simulink model "RIEKF_test"  (R2016b)
settings: Solver=ode23  StartTime=simulationParameters.startTime  StopTime=10  FixedStep=1e-5  EnableMultiTasking=on
InitFcn:
  | simulationInitFcn;
StartFcn:
  | simulationStartFcn;
StopFcn:
  | simulationStopFcn;
libraries: StateEstimation x1
settings Model: Creator=case  LastModifiedBy=Ross Hartley
settings SolverCC: EnableConcurrentExecution=on  ConcurrentTasks=on  ZeroCrossControl=DisableAll  InsertRTBMode=Always
settings DataIOCC: SaveOutput=off  SignalLogging=off  DSMLogging=off  SaveTime=off
settings OptimizationCC: DefaultParameterBehavior=Inlined  UseFloatMulNetSlope=on  InlineInvariantSignals=on  EfficientFloat2IntCast=on  LifeSpan=inf  SimCompilerOptimization=on  AccelVerboseBuild=on
settings DebuggingCC: ReadBeforeWriteMsg=DisableAll  WriteAfterWriteMsg=DisableAll  WriteAfterReadMsg=DisableAll  ParameterUnderflowMsg=error  ParameterTunabilityLossMsg=error  UniqueDataStoreMsg=error  AllowSymbolicDim=off  StrictBusMsg=ErrorOnBusTreatedAsVector  SFUnexpectedBacktrackingDiag=warning  SFNoUnconditionalDefaultTransitionDiag=warning  SFExecutionAtInitializationDiag=none
settings HardwareCC: TargetBitPerPointer=64  TargetBitPerSizeT=64  TargetBitPerPtrDiffT=64  TargetLongLongMode=on  TargetIntDivRoundTo=Zero  TargetEndianess=LittleEndian  TargetWordSize=64  TargetHWDeviceType=MATLAB Host  ProdEqTarget=off
settings ModelReferenceCC: UpdateModelReferenceTargets=IfOutOfDate  ModelReferenceNumInstancesAllowed=Zero  ModelReferenceMinAlgLoopOccurrences=on  PropagateSignalLabelsOutOfModel=off
settings RTWCC: RTWUseSimCustomCode=on  BuildConfiguration=Faster Runs  CheckMdlBeforeBuild=Warning
settings CodeAppCC: GenerateComments=off  SimulinkBlockComments=off
settings GRTTargetCC: MatFileLogging=off  MultiInstanceERTCode=on  CodeInterfacePackaging=Reusable function  SupportNonFinite=off  GenerateAllocFcn=on
settings ConfigComp: CovMetricSettings=dw  CovHtmlReporting=on  CovSaveCumulativeToWorkspaceVar=on  CovSaveSingleToWorkspaceVar=on  CovExternalEMLEnable=off
settings DiagnosticsConfigSet: SimMechanicsRigidlyBoundBlock=warning
settings ExplorerConfigSet: InternalSimMechanicsExplorerSettings="<ExplorerConfiguration><canonicalview>default</canonicalview><AnimationSetting><BasePlaybackSpeed>1.0</BasePlaybackSpeed><PlaybackSpeedFactor>1.0</PlaybackSpeedFactor></AnimationSetting><TilePanel><TileInfo><Tiles Columns=\"1\" Count=\"1\" Rows=\"1\"><Column Left=\"2\" Weight=\"1\"/><Column Left=\"1053\"/><Row Top=\"2\" Weight=\"1\"/><Row Top=\"486\"/><Tile Height=\"1\" Width=\"1\" X=\"0\" Y=\"0\"/></Tiles></TileInfo><SceneInfo><SceneViewer><BGColor><R>0.60000002384185791</R><G>0.60000002384185791</G><B>0.60000002384185791</B></BGColor><Camera><DoPerspective>on</DoPerspective><Position><X>1.5163613923952763</X><Y>-1.4988060678602755</Y><Z>0.66118837525886986</Z></Position><Center><X>0.016361392395276342</X><Y>0.0011939321397245184</Y><Z>0.16118837525886986</Z></Center><Up><X>0</X><Y>0</Y><Z>1</Z></Up><ViewLimDist>1</ViewLimDist><YLim>0.46630765815499858</YLim><XLim>1.0229317469421231</XLim></Camera></SceneViewer></SceneInfo></TilePanel><MechEditorPanel><Cameras><Camera><Id>Camera1</Id><Value><Name>Tracking Camera</Name><NativeCamera><PositionTrackingFeature>Cassie_V2_Simulation_Subsystem.Cassie_Multibody_Subsystem.Pelvis.Tracking_Camera.F</PositionTrackingFeature><CenterTrackingFeature>Cassie_V2_Simulation_Subsystem.Cassie_Multibody_Subsystem.Pelvis.Tracking_Camera_Target.F</CenterTrackingFeature><UpVectorTrackingFeature>Cassie_V2_Simulation_Subsystem.Cassie_Multibody_Subsystem.Pelvis.Tracking_Camera_Target.F</UpVectorTrackingFeature><CenterTrackingOrigin>on</CenterTrackingOrigin><UpVectorTrackingDirection>+Z</UpVectorTrackingDirection></NativeCamera></Value></Camera><Camera><Id>Camera2</Id><Value><Name>Fixed Camera</Name><NativeCamera><PositionTrackingFeature>Cassie_V2_Simulation_Subsystem.Cassie_Multibody_Subsystem.Pelvis.Fixed_Camera.F</PositionTrackingFeature><CenterTrackingFeature>Cassie_V2_Simulation_Subsystem.Cassie_Multibody_Subsystem.Pelvis.Fixed_Camera_Target.F</CenterTrackingFeature><UpVectorTrackingFeature>Cassie_V2_Simulation_Subsystem.Cassie_Multibody_Subsystem.Pelvis.Fixed_Camera_Target.F</UpVectorTrackingFeature><CenterTrackingOrigin>on</CenterTrackingOrigin><UpVectorTrackingDirection>+Z</UpVectorTrackingDirection></NativeCamera></Value></Camera></Cameras><GfxPanelCameraMap><MapElement CameraMLId=\"Camera1\" GfxPanelIndex=\"0\"/></GfxPanelCameraMap><VideoCreator><PlaybackSpeedRatio>1.0</PlaybackSpeedRatio><FrameRate>30</FrameRate><VideoFormat>Motion JPEG AVI</VideoFormat><FrameSize>auto</FrameSize></VideoCreator></MechEditorPanel></ExplorerConfiguration>"

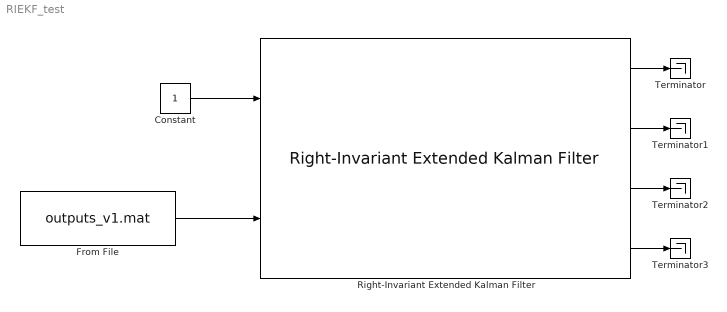
== system RIEKF_test ==
  Constant : Constant
  From File : FromFile  FileName=outputs_v1.mat  OutDataTypeStr=Bus: cassieOutputsBus  SampleTime=0
  Right-Invariant Extended Kalman Filter : StateEstimation/Right-Invariant Extended Kalman Filter  SimulationMode=Normal  CodeInterface=Model reference  ModelReferenceVersion=1.1360
  Terminator{,1..3} (4 alike) : Terminator
  wires:
  From File/1 -> Right-Invariant Extended Kalman Filter/2
  Constant/1 -> Right-Invariant Extended Kalman Filter/1
  Right-Invariant Extended Kalman Filter/1 -> Terminator/1
  Right-Invariant Extended Kalman Filter/2 -> Terminator1/1
  Right-Invariant Extended Kalman Filter/3 -> Terminator2/1
  Right-Invariant Extended Kalman Filter/4 -> Terminator3/1
